simulink model "Ampliutde_Modulation_Based_On_Block_Diagrams"  (R2013a)
settings: Solver=ode45  StartTime=0.0  StopTime=3e-3  MaxStep=0.001e-3  RelTol=1e-3
settings Model: Creator=B407  LastModifiedBy=B407

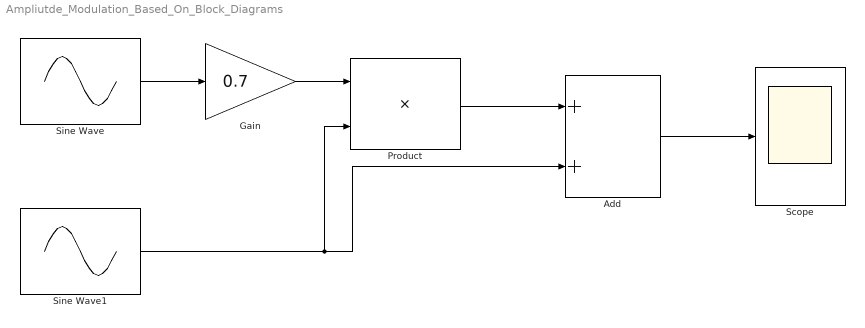
== system Ampliutde_Modulation_Based_On_Block_Diagrams ==
  Add : Sum
  Gain : Gain  Gain=0.7
  Product : Product
  Scope : Scope
  Sine Wave : Sin  Frequency=6280  Phase=3.14/2  SampleTime=0
  Sine Wave1 : Sin  Frequency=20*6280  Phase=3.14/2  SampleTime=0
  wires:
  Sine Wave/1 -> Gain/1
  Gain/1 -> Product/1
  Sine Wave1/1 -> Product/2, Add/2
  Product/1 -> Add/1
  Add/1 -> Scope/1
